simulink model "lv_windturbine"  (Simulink 7.1)
settings: Solver=ode45  StartTime=0.0  StopTime=10.0  RelTol=1e-3
libraries: DRlib x1
settings Model: Creator=lv  LastModifiedBy=lv

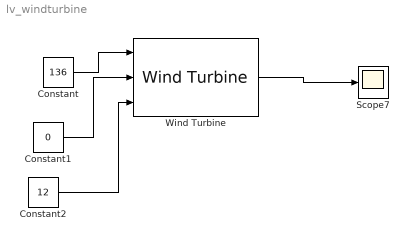
== system lv_windturbine ==
  Constant : Constant  Value=136  OutDataType=sfix(16)  OutScaling=2^0
  Constant1 : Constant  Value=0  OutDataType=sfix(16)  OutScaling=2^0
  Constant2 : Constant  Value=12  OutDataType=sfix(16)  OutScaling=2^0
  Scope7 : Scope
      settings: TimeRange=50  YMin=0.1772981595092024  YMax=0.2028981595092024
  Wind Turbine : DRlib/Wind Generation/Wind Turbine  DialogController=POWERSYS.PowerSysDialog  SystemSampleTime=-1  Pnom=1.5e6  Pelec_base=1.5e6/0.9  wind_base=12  P_wind_base=0.73  speed_nom=1.2  pitch_angle=0  DisplayTurbChar=off  c1_c6="[0.51763          116          0.4            5           21     0.006795]"  cp_nom=0.48  lambda_nom=8.1
  wires:
  Wind Turbine/1 -> Scope7/1
  Constant/1 -> Wind Turbine/1
  Constant1/1 -> Wind Turbine/2
  Constant2/1 -> Wind Turbine/3
